simulink model "MFinal"  (R2024b)
settings: configuration reference "STM32H7_Config" (kept outside this file)
settings Model: DataDictionary=Master_Dictionary.sldd  EnableAccessToBaseWorkspace=off  Creator=torni  LastModifiedBy=Will
settings ConfigSetRef: SourceName=STM32H7_Config

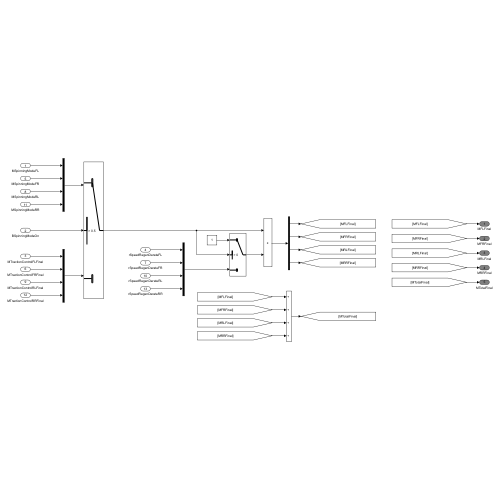
[thumbnail: Simulink's stored preview of the top-level diagram]
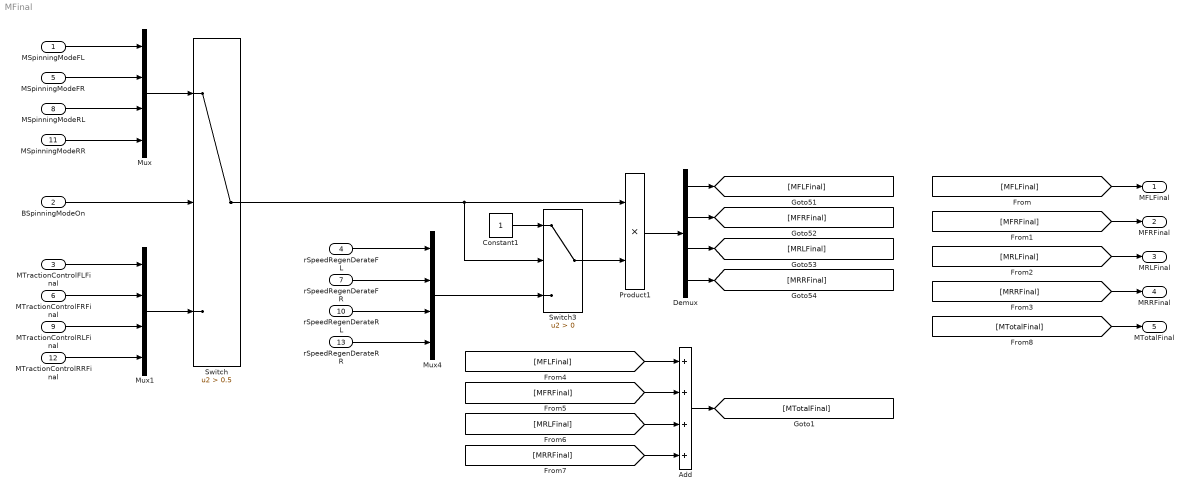
== system MFinal ==
  MSpinningModeFL : Inport
  BSpinningModeOn : Inport  Port=2  OutDataTypeStr=boolean
  MTractionControlFLFinal : Inport  Port=3
  rSpeedRegenDerateFL : Inport  Port=4
  MSpinningModeFR : Inport  Port=5
  MTractionControlFRFinal : Inport  Port=6
  rSpeedRegenDerateFR : Inport  Port=7
  MSpinningModeRL : Inport  Port=8
  MTractionControlRLFinal : Inport  Port=9
  rSpeedRegenDerateRL : Inport  Port=10
  MSpinningModeRR : Inport  Port=11
  MTractionControlRRFinal : Inport  Port=12
  rSpeedRegenDerateRR : Inport  Port=13
  Add : Sum  Inputs=++++
  Constant1 : Constant
  Demux : Demux
  Mux : Mux
  Mux1 : Mux
  Mux4 : Mux
  Product1 : Product
  Switch : Switch  Criteria=u2 > Threshold  Threshold=0.5  SaturateOnIntegerOverflow=off  InputSameDT=off
  Switch3 : Switch  Criteria=u2 > Threshold  SaturateOnIntegerOverflow=off  InputSameDT=off
  MFLFinal : Outport  OutDataTypeStr=double  VectorParamsAs1DForOutWhenUnconnected=off
  MFRFinal : Outport  Port=2  OutDataTypeStr=double  VectorParamsAs1DForOutWhenUnconnected=off
  MRLFinal : Outport  Port=3  OutDataTypeStr=double  VectorParamsAs1DForOutWhenUnconnected=off
  MRRFinal : Outport  Port=4  OutDataTypeStr=double  VectorParamsAs1DForOutWhenUnconnected=off
  MTotalFinal : Outport  Port=5  OutDataTypeStr=double  VectorParamsAs1DForOutWhenUnconnected=off
  wires:
  [MFLFinal] -> MFLFinal/1
  [MFRFinal] -> MFRFinal/1
  [MRLFinal] -> MRLFinal/1
  [MRRFinal] -> MRRFinal/1
  Add/1 -> [MTotalFinal]
  [MTotalFinal] -> MTotalFinal/1
  MSpinningModeFL/1 -> Mux/1
  MSpinningModeFR/1 -> Mux/2
  MSpinningModeRL/1 -> Mux/3
  MSpinningModeRR/1 -> Mux/4
  Mux/1 -> Switch/1
  BSpinningModeOn/1 -> Switch/2
  Mux1/1 -> Switch/3
  MTractionControlFLFinal/1 -> Mux1/1
  MTractionControlFRFinal/1 -> Mux1/2
  MTractionControlRLFinal/1 -> Mux1/3
  MTractionControlRRFinal/1 -> Mux1/4
  Constant1/1 -> Switch3/1
  Switch/1 -> Switch3/2, Product1/1
  rSpeedRegenDerateFR/1 -> Mux4/2
  rSpeedRegenDerateFL/1 -> Mux4/1
  Mux4/1 -> Switch3/3
  rSpeedRegenDerateRL/1 -> Mux4/3
  rSpeedRegenDerateRR/1 -> Mux4/4
  Product1/1 -> Demux/1
  Switch3/1 -> Product1/2
  Demux/1 -> [MFLFinal]
  Demux/2 -> [MFRFinal]
  Demux/3 -> [MRLFinal]
  Demux/4 -> [MRRFinal]
  [MFLFinal] -> Add/1
  [MFRFinal] -> Add/2
  [MRRFinal] -> Add/4
  [MRLFinal] -> Add/3
